simulink model "FindLimits2020b"  (R2021b)
settings: Solver=FixedStepDiscrete  StartTime=0.0  StopTime=inf  RelTol=1e-3  EnableMultiTasking=on
values from neighbouring files (symbols this model uses):
  duty_max = 0.9    [Parameters.m]
  duty_min = 0    [Parameters.m]
  potentiometer_max = 1.0    (= 1)    [Parameters.m]
  potentiometer_min = 0.3    [Parameters.m]
libraries: ec_arm_cortex_a_lib x5
settings Model: SimulationMode=external  Creator=Lab_Auto  LastModifiedBy=barag
settings SolverCC: AlgebraicLoopSolver=TrustRegion  PositivePriorityOrder=on
settings DataIOCC: LimitDataPoints=on  ReturnWorkspaceOutputs=off
settings OptimizationCC: LifeSpan=Inf  MaxStackSize=64  EfficientTunableParamExpr=on
settings DebuggingCC: AllowSymbolicDim=off  SFUnexpectedBacktrackingDiag=warning  SFNoUnconditionalDefaultTransitionDiag=warning  SFExecutionAtInitializationDiag=none  SFMachineParentedDataDiag=warning  ArithmeticOperatorsInVariantConditions=warning
settings HardwareCC: ProdBitPerPointer=32  ProdBitPerSizeT=32  ProdBitPerPtrDiffT=32  ProdLargestAtomicInteger=Long  ProdLargestAtomicFloat=Double  ProdWordSize=32  ProdHWDeviceType=ARM Compatible->ARM Cortex
settings ModelReferenceCC: PropagateSignalLabelsOutOfModel=off
settings SFSimCC: SimUseLocalCustomCode=off  MATLABDynamicMemAlloc=off  CustomCodeUndefinedFunction=UseInterfaceOnly
settings RTWCC: Description=Embedded Coder  SystemTargetFile=ert.tlc  HardwareBoard=BeagleBone Black  TLCOptions=-aInlineSetEventsForThisBaseRateFcn=TLC_FALSE -aSuppressMultiTaskScheduler=TLC_FALSE -aRateBasedStepFcn=0  TemplateMakefile=ert_default_tmf  RTWUseLocalCustomCode=off  Toolchain=Linaro Toolchain v4.8
settings CodeAppCC: IgnoreCustomStorageClasses=off  StateflowObjectComments=on
settings ERTTargetCC: MultiwordLength=2048  ConvertIfToSwitch=off  SuppressUnreachableDefaultCases=off
settings ConfigComp: CovMetricSettings=dw  CovSaveCumulativeToWorkspaceVar=on  CovSaveSingleToWorkspaceVar=on  CovExternalEMLEnable=off

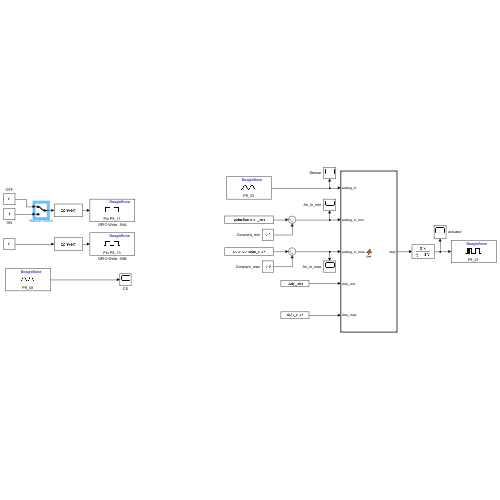
[thumbnail: Simulink's stored preview of the top-level diagram]
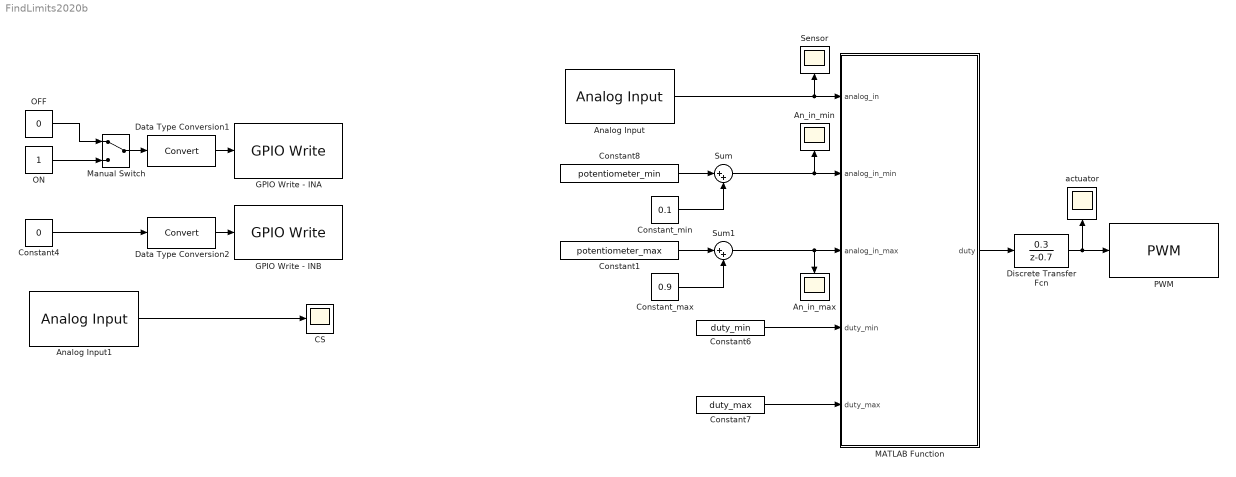
== system FindLimits2020b ==
  " OFF" : Constant  Value=0
  An_in_max : Scope
  An_in_min : Scope
  Analog Input : ec_arm_cortex_a_lib/Analog Input  board=BeagleBone Black  pin=P9_33  sampleTime=0.01  blockPlatform=BeagleBone
      settings: SourceProductBaseCode=ECCORTEXA
  Analog Input1 : ec_arm_cortex_a_lib/Analog Input  board=BeagleBone Black  pin=P9_40  sampleTime=0.01  blockPlatform=BeagleBone
      settings: SourceProductBaseCode=ECCORTEXA
  CS : Scope
  Constant1 : Constant  Value=potentiometer_max
  Constant4 : Constant  Value=0
  Constant6 : Constant  Value=duty_min
  Constant7 : Constant  Value=duty_max
  Constant8 : Constant  Value=potentiometer_min
  Constant_max : Constant  Value=0.9
  Constant_min : Constant  Value=0.1
  Data Type Conversion1 : DataTypeConversion
  Data Type Conversion2 : DataTypeConversion
  Discrete Transfer Fcn : DiscreteTransferFcn  Numerator=[0.3]  Denominator=[1 -0.7]
  GPIO Write - INA : ec_arm_cortex_a_lib/GPIO Write  board=BeagleBone Black  gpio=P9_11  direction=Output  blockPlatform=BeagleBone
      settings: SourceProductBaseCode=ECCORTEXA
  GPIO Write - INB : ec_arm_cortex_a_lib/GPIO Write  board=BeagleBone Black  gpio=P9_13  direction=Output  blockPlatform=BeagleBone
      settings: SourceProductBaseCode=ECCORTEXA
  MATLAB Function : MATLAB Function  TreatAsAtomicUnit=on
  Manual Switch : ManualSwitch
  ON : Constant
  PWM : ec_arm_cortex_a_lib/PWM  board=BeagleBone Black  pin=P9_21  frequency=20000  polarity=Positive  blockPlatform=BeagleBone
      settings: SourceProductBaseCode=ECCORTEXA
  Sensor : Scope
  Sum : Sum  Inputs=|++
  Sum1 : Sum  Inputs=|++
  actuator : Scope
  wires:
  Analog Input1/1 -> CS/1
  Data Type Conversion1/1 -> GPIO Write - INA/1
  Sum/1 -> MATLAB Function/2(analog_in_min), An_in_min/1
  Constant_max/1 -> Sum1/2
  MATLAB Function/1(duty) -> Discrete Transfer Fcn/1
  Constant8/1 -> Sum/1
  Analog Input/1 -> MATLAB Function/1(analog_in), Sensor/1
  " OFF"/1 -> Manual Switch/1
  Constant6/1 -> MATLAB Function/4(duty_min)
  Constant7/1 -> MATLAB Function/5(duty_max)
  ON/1 -> Manual Switch/2
  Data Type Conversion2/1 -> GPIO Write - INB/1
  Constant_min/1 -> Sum/2
  Discrete Transfer Fcn/1 -> PWM/1, actuator/1
  Sum1/1 -> MATLAB Function/3(analog_in_max), An_in_max/1
  Manual Switch/1 -> Data Type Conversion1/1
  Constant1/1 -> Sum1/1
  Constant4/1 -> Data Type Conversion2/1

== matlab function FindLimits2020b/MATLAB Function ==
  data: analog_in input; duty output; analog_in_min input; analog_in_max input; duty_min input; duty_max input
function duty= fcn(analog_in, analog_in_min, analog_in_max, duty_min, duty_max)
%#codegen
persistent flag;


if isempty(flag)
    flag = 0;
end

duty = duty_min;

if flag == 0
    duty = duty_min;
    if (flag == 0) && (analog_in <= analog_in_min)
        flag = 1;
        duty = duty_max;
    end
end

if flag == 1
    duty = duty_max;
    if (flag == 1) && (analog_in >= analog_in_max)
        flag = 0;
        duty = duty_min;
    end
end
